simulink model "clik_inverse"  (Simulink 10.2)
settings: Solver=ode1  StartTime=0.0  StopTime=4  FixedStep=0.001  RelTol=1e-3
undefined symbols (not defined in the file or in its folder): DiscIntNeverNeededParam, q0, Tc
settings Model: Creator=Xp  LastModifiedBy=venkygoka
settings DataIOCC: LimitDataPoints=on
settings OptimizationCC: ExpressionDepthLimit=2147483647  InitFltsAndDblsToZero=on
settings DebuggingCC: SaveWithParameterizedLinksMsg=none  SolverPrmCheckMsg=warning  MultiTaskDSMMsg=warning  MultiTaskCondExecSysMsg=none  StateNameClashWarn=warning
settings SFSimCC: SimUseLocalCustomCode=on
settings RTWCC: RTWUseLocalCustomCode=on
settings ConfigComp: CovExternalEMLEnable=on

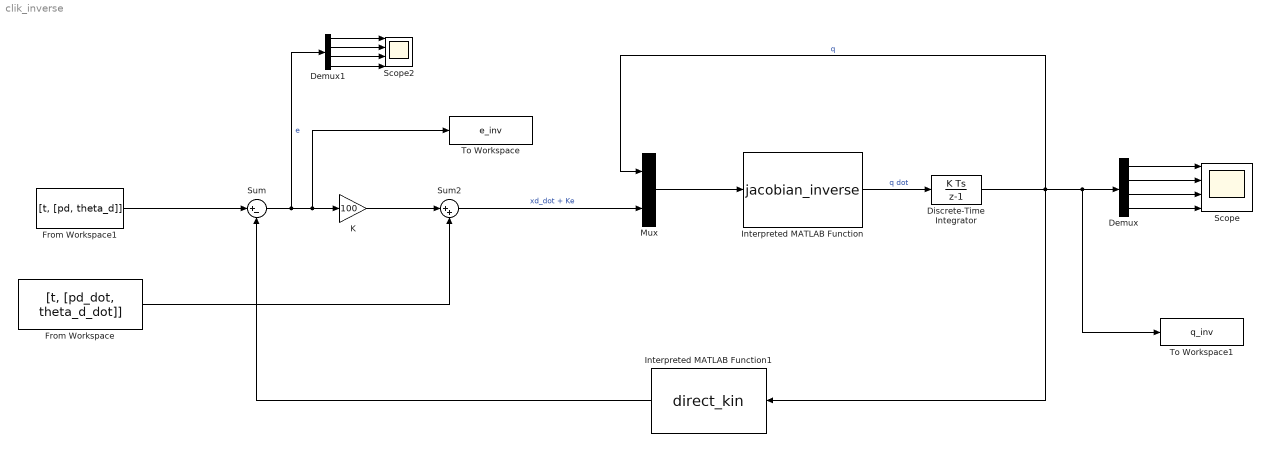
== system clik_inverse ==
  Demux : Demux
  Demux1 : Demux
  Discrete-Time Integrator : DiscreteIntegrator  InitialCondition=q0  SampleTime=Tc  LimitOutput=on  UpperSaturationLimit=[pi/2, pi/4, 1, 2*pi]  LowerSaturationLimit=[-pi/2, -pi/2, 0.25, -2*pi]  ICPrevOutput=DiscIntNeverNeededParam  ICPrevScaledInput=DiscIntNeverNeededParam
  From Workspace : FromWorkspace  VariableName=[t, [pd_dot, theta_d_dot]]
  From Workspace1 : FromWorkspace  VariableName=[t, [pd, theta_d]]
  Interpreted MATLAB Function : MATLABFcn  MATLABFcn=jacobian_inverse
  Interpreted MATLAB Function1 : MATLABFcn  MATLABFcn=direct_kin
  K : Gain  Gain=100
  Mux : Mux  Inputs=2
  Scope : Scope  NumInputPorts=4
  Scope2 : Scope  NumInputPorts=4
  Sum : Sum  Inputs=|+-
  Sum2 : Sum  Inputs=|++
  To Workspace : ToWorkspace  VariableName=e_inv  SaveFormat=Timeseries  SampleTime=-1
  To Workspace1 : ToWorkspace  VariableName=q_inv  SaveFormat=Timeseries  SampleTime=-1
  wires:
  Sum/1 -> Demux1/1, To Workspace/1, K/1  "e"
  K/1 -> Sum2/1
  Sum2/1 -> Mux/2  "xd_dot + Ke"
  Discrete-Time Integrator/1 -> Interpreted MATLAB Function1/1, Mux/1, To Workspace1/1, Demux/1  "q"
  Interpreted MATLAB Function/1 -> Discrete-Time Integrator/1  "q dot"
  From Workspace1/1 -> Sum/1
  Interpreted MATLAB Function1/1 -> Sum/2
  From Workspace/1 -> Sum2/2
  Demux/1 -> Scope/1
  Demux/2 -> Scope/2
  Demux/3 -> Scope/3
  Demux/4 -> Scope/4
  Mux/1 -> Interpreted MATLAB Function/1
  Demux1/4 -> Scope2/4
  Demux1/3 -> Scope2/3
  Demux1/2 -> Scope2/2
  Demux1/1 -> Scope2/1
